simulink model "sensorSimulation"  (Simulink 7.5)
settings: Solver=ode8  StartTime=0.0  StopTime=5e-3  RelTol=1e-9  AbsTol=1e-9
values from neighbouring files (symbols this model uses):
  k = self.k_mo    [cantilever.m]
undefined symbols (not defined in the file or in its folder): b, Kamp, m, SFpr, Sfv, Tamp, Thighpass, Tlowpass
settings Model: Creator=jcdoll  LastModifiedBy=jcdoll
settings SolverCC: InitialStep=1e-7  ZeroCrossAlgorithm=Adaptive
settings DataIOCC: TimeSaveName=time
settings OptimizationCC: InitFltsAndDblsToZero=on
settings DebuggingCC: SolverPrmCheckMsg=none  StrictBusMsg=Warning

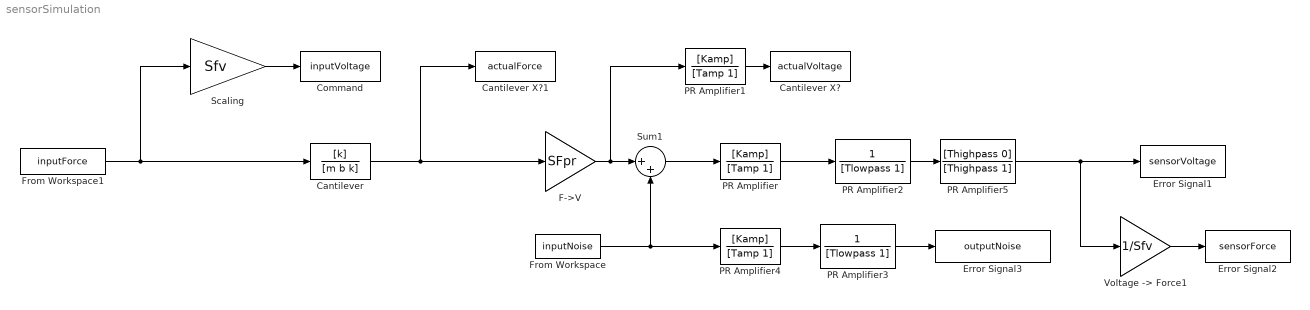
== system sensorSimulation ==
  Cantilever : TransferFcn  Numerator=[k]  Denominator=[m b k]
  Cantilever X? : ToWorkspace  VariableName=actualVoltage  SampleTime=-1  SaveFormat=Array
  Cantilever X?1 : ToWorkspace  VariableName=actualForce  SampleTime=-1  SaveFormat=Array
  Command : ToWorkspace  VariableName=inputVoltage  SampleTime=-1  SaveFormat=Array
  Error Signal1 : ToWorkspace  VariableName=sensorVoltage  SampleTime=-1  SaveFormat=Array
  Error Signal2 : ToWorkspace  VariableName=sensorForce  SampleTime=-1  SaveFormat=Array
  Error Signal3 : ToWorkspace  VariableName=outputNoise  SampleTime=-1  SaveFormat=Array
  F->V : Gain  Gain=SFpr  ParameterDataType=sfix(16)  ParameterScaling=2^0  OutDataType=sfix(16)  OutScaling=2^0
  From Workspace : FromWorkspace  VariableName=inputNoise  SampleTime=0
  From Workspace1 : FromWorkspace  VariableName=inputForce  SampleTime=0
  PR Amplifier : TransferFcn  Numerator=[Kamp]  Denominator=[Tamp 1]
  PR Amplifier1 : TransferFcn  Numerator=[Kamp]  Denominator=[Tamp 1]
  PR Amplifier2 : TransferFcn  Numerator=1  Denominator=[Tlowpass 1]
  PR Amplifier3 : TransferFcn  Numerator=1  Denominator=[Tlowpass 1]
  PR Amplifier4 : TransferFcn  Numerator=[Kamp]  Denominator=[Tamp 1]
  PR Amplifier5 : TransferFcn  Numerator=[Thighpass 0]  Denominator=[Thighpass 1]
  Scaling : Gain  Gain=Sfv  ParameterDataType=sfix(16)  ParameterScaling=2^0  OutDataType=sfix(16)  OutScaling=2^0
  Sum1 : Sum  Inputs=|++  OutDataType=sfix(16)  OutScaling=2^0
  "Voltage -> Force1" : Gain  Gain=1/Sfv  ParameterDataType=sfix(16)  ParameterScaling=2^0  OutDataType=sfix(16)  OutScaling=2^0
  wires:
  Cantilever/1 -> Cantilever X?1/1, F->V/1
  From Workspace/1 -> Sum1/2, PR Amplifier4/1
  "Voltage -> Force1"/1 -> Error Signal2/1
  Scaling/1 -> Command/1
  From Workspace1/1 -> Scaling/1, Cantilever/1
  F->V/1 -> Sum1/1, PR Amplifier1/1
  PR Amplifier1/1 -> Cantilever X?/1
  PR Amplifier/1 -> PR Amplifier2/1
  Sum1/1 -> PR Amplifier/1
  PR Amplifier4/1 -> PR Amplifier3/1
  PR Amplifier3/1 -> Error Signal3/1
  PR Amplifier2/1 -> PR Amplifier5/1
  PR Amplifier5/1 -> Error Signal1/1, "Voltage -> Force1"/1
